simulink model "simulink"  (R2017a)
settings: Solver=ode5  StartTime=0.0  StopTime=inf  FixedStep=SampleTime  RelTol=1e-3  EnableMultiTasking=on
values from neighbouring files (symbols this model uses):
  max_velocity_1 = 14    [Matlab_script.m]
  max_velocity_2 = 15    [Matlab_script.m]
  max_velocity_3 = 13    [Matlab_script.m]
  max_velocity_4 = 100    [Matlab_script.m]
  SampleTime = 0.002    [Matlab_script.m]
  XY_vel = 0.5    [Matlab_script.m]
libraries: xpcrtudplib x2, etargetslib x1, xpcutilitieslib x1
settings Model: Creator=kivela6  LastModifiedBy=bangalor
settings SolverCC: EnableConcurrentExecution=on  ConcurrentTasks=on  AutoInsertRateTranBlk=on
settings DataIOCC: LimitDataPoints=on  SaveFormat=StructureWithTime  SignalLoggingSaveFormat=ModelDataLogs
settings OptimizationCC: BlockReduction=off  OptimizeBlockIOStorage=off  BufferReuse=off  GlobalBufferReuse=off  ExpressionFolding=off  EnableMemcpy=off  ExpressionDepthLimit=2147483647  LocalBlockOutputs=off
settings DebuggingCC: UnderspecifiedInitializationDetection=Classic  MergeDetectMultiDrivingBlocksExec=none  SolverPrmCheckMsg=warning  FcnCallInpInsideContextMsg=warning  StateNameClashWarn=warning  SFUnexpectedBacktrackingDiag=warning  SFNoUnconditionalDefaultTransitionDiag=warning  SFExecutionAtInitializationDiag=none
settings HardwareCC: ProdBitPerPointer=32  ProdBitPerSizeT=32  ProdBitPerPtrDiffT=32  ProdLargestAtomicFloat=None  ProdWordSize=32  ProdLongLongMode=on  ProdHWDeviceType=Generic->32-bit x86 compatible
settings ModelReferenceCC: PropagateSignalLabelsOutOfModel=off
settings RTWCC: SystemTargetFile=slrt.tlc  TemplateMakefile=slrt_default_tmf  Description=Simulink Real-Time  RTWCompilerOptimization=on
settings SimulinkRealTimeCC: xPCisDownloadable=off  xPCConcurrentTasks=on
settings ConfigComp: CovMetricSettings=dw  CovHtmlReporting=on  CovSaveCumulativeToWorkspaceVar=on  CovSaveSingleToWorkspaceVar=on  CovExternalEMLEnable=off  CovSFcnEnable=off

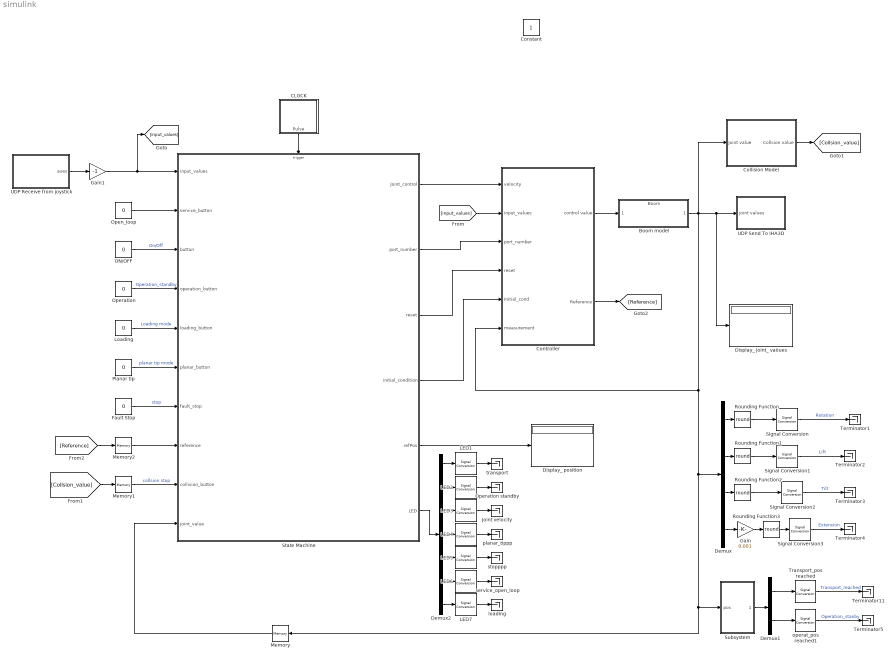
== system simulink ==
  Boom model : ModelReference  ModelNameDialog=Boom.slxp  ModelReferenceVersion=1.513  CopyOfModelProtected=on
  CLOCK : Subsystem
  Collision Model : Subsystem
  Controller : Subsystem
  Demux : Demux
  Demux1 : Demux  Outputs=2
  Demux2 : Demux  Outputs=7
  Display_ joint_ vaöues : Display
  Display_ position : Display
  Fault Stop : Constant  Value=0
  Gain : Gain  Gain=0.001
  Gain1 : Gain  Gain=-1
  Joint velocity : Terminator
  LED{1..7} (7 alike) : SignalConversion  OverrideOpt=off
  Loading : Constant  Value=0
  Memory : Memory
  Memory1 : Memory
  Memory2 : Memory
  ON/OFF : Constant  Value=0
  Open_loop : Constant  Value=0
  Operation : Constant  Value=0
  Operation standby : Terminator
  Planar tip : Constant  Value=0
  Rounding Function{,1..3} (4 alike) : Rounding  Operator=round
  Signal Conversion{,1..3} (4 alike) : SignalConversion  OverrideOpt=off
  State Machine : Stateflow chart  TreatAsAtomicUnit=on
  Subsystem : Subsystem
  Terminator{1..5,11} (6 alike) : Terminator
  Transport_pos reached : SignalConversion  OverrideOpt=off
  UDP Receive from joystick : Subsystem
  UDP Send To IHA3D : Subsystem
  loading : Terminator
  operat_pos reached1 : SignalConversion  OverrideOpt=off
  planar_tippp : Terminator
  service_open_loop : Terminator
  stopppp : Terminator
  transport : Terminator
  Constant : Constant  IOType=siggen
  wires:
  State Machine/1(Joint_control) -> Controller/1(velocity)
  CLOCK/1(Pulse) -> State Machine/Trigger
  Controller/1(control value) -> Boom model/1
  Memory/1 -> State Machine/10(joint_value)
  [input_values] -> Controller/2(input_values)
  State Machine/2(port_number) -> Controller/3(port_number)
  State Machine/3(reset) -> Controller/4(reset)
  State Machine/4(initial_condition) -> Controller/5(Initial_cond)
  Demux/1 -> Rounding Function/1
  Rounding Function/1 -> Signal Conversion/1
  Signal Conversion/1 -> Terminator1/1  "Rotation"
  Signal Conversion1/1 -> Terminator2/1  "Lift"
  Rounding Function1/1 -> Signal Conversion1/1
  Demux/2 -> Rounding Function1/1
  Demux/3 -> Rounding Function2/1
  Rounding Function2/1 -> Signal Conversion2/1
  Signal Conversion2/1 -> Terminator3/1  "Tilt"
  Signal Conversion3/1 -> Terminator4/1  "Extension"
  ON/OFF/1 -> State Machine/3(button)  "On/Off"
  Operation/1 -> State Machine/4(operation_button)  "Operation_standby"
  Loading/1 -> State Machine/5(loading_button)  "Loading mode"
  Planar tip/1 -> State Machine/6(planar_button)  "planar tip mode"
  Collision Model/1(Collsion value) -> [Collsion_value]
  UDP Receive from joystick/1(axes) -> Gain1/1
  Open_loop/1 -> State Machine/2(service_button)
  [Collsion_value] -> Memory1/1
  Fault Stop/1 -> State Machine/7(fault_stop)  "stop"
  Memory1/1 -> State Machine/9(collision_button)  "collsion stop"
  State Machine/5(refPos) -> Display_ position/1
  Demux1/2 -> operat_pos reached1/1
  Demux1/1 -> Transport_pos reached/1
  Boom model/1 -> Display_ joint_ vaöues/1, UDP Send To IHA3D/1(joint values), Controller/6(measurement), Memory/1, Subsystem/1(pos), Demux/1, Collision Model/1(Joint value)
  Subsystem/1(LED State) -> Demux1/1
  Transport_pos reached/1 -> Terminator11/1  "Transport_reached"
  State Machine/6(LED) -> Demux2/1
  Demux2/1 -> LED1/1
  LED1/1 -> transport/1
  LED2/1 -> Operation standby/1
  Demux2/2 -> LED2/1
  LED3/1 -> Joint velocity/1
  Demux2/3 -> LED3/1
  LED4/1 -> planar_tippp/1
  Demux2/4 -> LED4/1
  LED5/1 -> stopppp/1
  Demux2/5 -> LED5/1
  LED6/1 -> service_open_loop/1
  Demux2/6 -> LED6/1
  Demux2/7 -> LED7/1
  operat_pos reached1/1 -> Terminator5/1  "Operation_stanby"
  Controller/2(Reference) -> [Reference]
  [Reference] -> Memory2/1
  Memory2/1 -> State Machine/8(reference)
  LED7/1 -> loading/1
  Gain/1 -> Rounding Function3/1
  Rounding Function3/1 -> Signal Conversion3/1
  Demux/4 -> Gain/1
  Gain1/1 -> [input_values], State Machine/1(input_values)

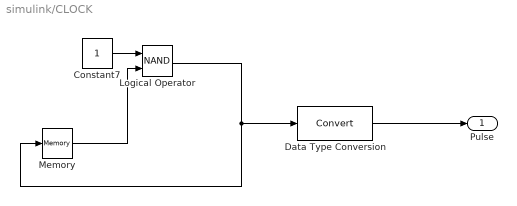
== system simulink/CLOCK ==
  Constant7 : Constant
  Data Type Conversion : DataTypeConversion
  Logical Operator : Logic  Operator=NAND  AllPortsSameDT=off  OutDataTypeStr=boolean
  Memory : Memory
  Pulse : Outport
  wires:
  Memory/1 -> Logical Operator/2
  Constant7/1 -> Logical Operator/1
  Logical Operator/1 -> Memory/1, Data Type Conversion/1
  Data Type Conversion/1 -> Pulse/1

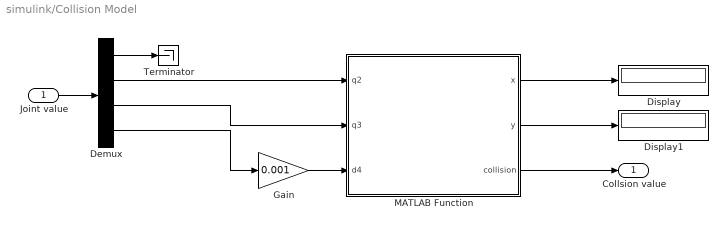
== system simulink/Collision Model ==
  Joint value : Inport
  Demux : Demux
  Display : Display
  Display1 : Display
  Gain : Gain  Gain=0.001
  MATLAB Function : MATLAB Function  TreatAsAtomicUnit=on
  Terminator : Terminator
  Collsion value : Outport
  wires:
  Demux/4 -> Gain/1
  MATLAB Function/2(y) -> Display1/1
  MATLAB Function/1(x) -> Display/1
  MATLAB Function/3(collision) -> Collsion value/1
  Demux/3 -> MATLAB Function/2(q3)
  Demux/2 -> MATLAB Function/1(q2)
  Demux/1 -> Terminator/1
  Joint value/1 -> Demux/1
  Gain/1 -> MATLAB Function/3(d4)

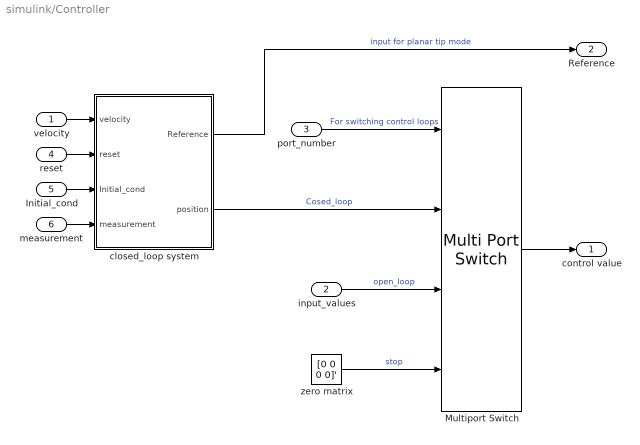
== system simulink/Controller ==
  velocity : Inport
  input_values : Inport  Port=2
  port_number : Inport  Port=3
  reset : Inport  Port=4
  Initial_cond : Inport  Port=5
  measurement : Inport  Port=6
  Multiport Switch : MultiPortSwitch  DiagnosticForDefault=Warning
  closed_loop system : Subsystem
  zero matrix : Constant  Value=[0 0 0 0]'
  control value : Outport
  Reference : Outport  Port=2
  wires:
  zero matrix/1 -> Multiport Switch/4  "stop"
  Multiport Switch/1 -> control value/1
  input_values/1 -> Multiport Switch/3  "open_loop"
  port_number/1 -> Multiport Switch/1  "For switching control loops"
  velocity/1 -> closed_loop system/1(velocity)
  reset/1 -> closed_loop system/2(reset)
  Initial_cond/1 -> closed_loop system/3(Initial_cond)
  measurement/1 -> closed_loop system/4(measurement)
  closed_loop system/1(Reference) -> Reference/1  "input for planar tip mode"
  closed_loop system/2(position) -> Multiport Switch/2  "Cosed_loop"

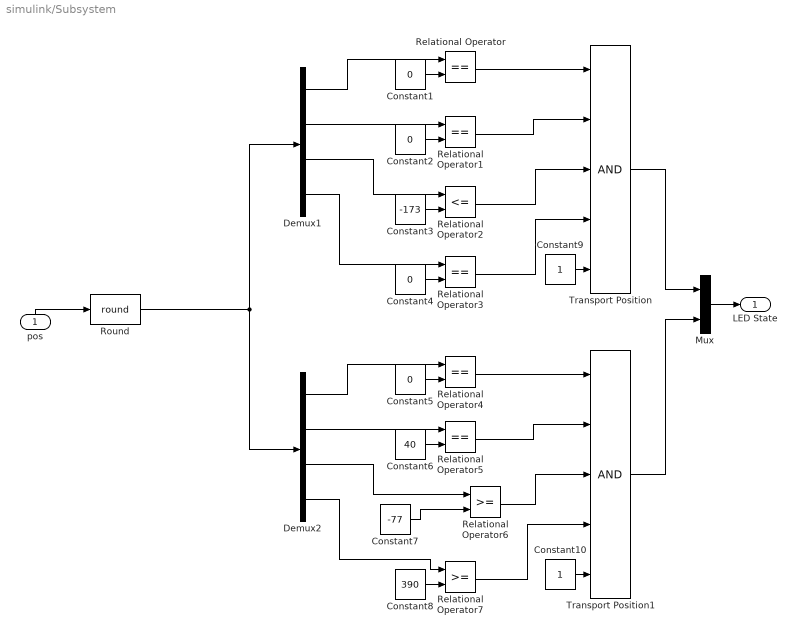
== system simulink/Subsystem ==
  pos : Inport
  Constant{1..2,4..5} (4 alike) : Constant  Value=0
  Constant10 : Constant
  Constant3 : Constant  Value=-173
  Constant6 : Constant  Value=40
  Constant7 : Constant  Value=-77
  Constant8 : Constant  Value=390
  Constant9 : Constant
  Demux1 : Demux
  Demux2 : Demux
  Mux : Mux  Inputs=2
  Relational Operator{,1,3..5} (5 alike) : RelationalOperator  Operator===  OutDataTypeStr=boolean  RndMeth=Simplest
  Relational Operator2 : RelationalOperator  Operator=<=  OutDataTypeStr=boolean  RndMeth=Simplest
  Relational Operator6 : RelationalOperator  OutDataTypeStr=boolean  RndMeth=Simplest
  Relational Operator7 : RelationalOperator  OutDataTypeStr=boolean  RndMeth=Simplest
  Round : Rounding  Operator=round
  Transport Position : Logic  Inputs=5  AllPortsSameDT=off  OutDataTypeStr=boolean
  Transport Position1 : Logic  Inputs=5  AllPortsSameDT=off  OutDataTypeStr=boolean
  LED State : Outport
  wires:
  Demux1/4 -> Relational Operator3/1
  Relational Operator3/1 -> Transport Position/4
  Constant4/1 -> Relational Operator3/2
  pos/1 -> Round/1
  Constant9/1 -> Transport Position/5
  Relational Operator4/1 -> Transport Position1/1
  Relational Operator5/1 -> Transport Position1/2
  Relational Operator7/1 -> Transport Position1/4
  Constant10/1 -> Transport Position1/5
  Relational Operator6/1 -> Transport Position1/3
  Relational Operator/1 -> Transport Position/1
  Constant1/1 -> Relational Operator/2
  Transport Position/1 -> Mux/1
  Relational Operator2/1 -> Transport Position/3
  Relational Operator1/1 -> Transport Position/2
  Demux2/1 -> Relational Operator4/1
  Demux2/2 -> Relational Operator5/1
  Constant8/1 -> Relational Operator7/2
  Demux2/3 -> Relational Operator6/1
  Constant5/1 -> Relational Operator4/2
  Constant6/1 -> Relational Operator5/2
  Demux2/4 -> Relational Operator7/1
  Constant2/1 -> Relational Operator1/2
  Constant3/1 -> Relational Operator2/2
  Demux1/3 -> Relational Operator2/1
  Demux1/2 -> Relational Operator1/1
  Demux1/1 -> Relational Operator/1
  Transport Position1/1 -> Mux/2
  Mux/1 -> LED State/1
  Round/1 -> Demux1/1, Demux2/1
  Constant7/1 -> Relational Operator6/2

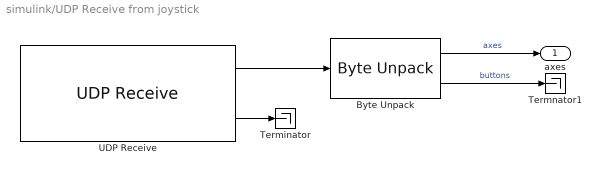
== system simulink/UDP Receive from joystick ==
  Byte Unpack : etargetslib/Byte Unpack  dimensions={4,12}  datatypes={'double','uint8'}  byteAlign=1
  Terminator : Terminator
  Termnator1 : Terminator
  UDP Receive : xpcrtudplib/UDP Receive  ipAddressVal=Use host-target connection  localPort=55550  rcvWidth=44  rcvFmAny=off  fmAddress=192.168.10.1  sampleTime=-1
      settings: SourceProductName=Simulink Real-Time
  axes : Outport
  wires:
  UDP Receive/2 -> Terminator/1
  UDP Receive/1 -> Byte Unpack/1
  Byte Unpack/1 -> axes/1  "axes"
  Byte Unpack/2 -> Termnator1/1  "buttons"

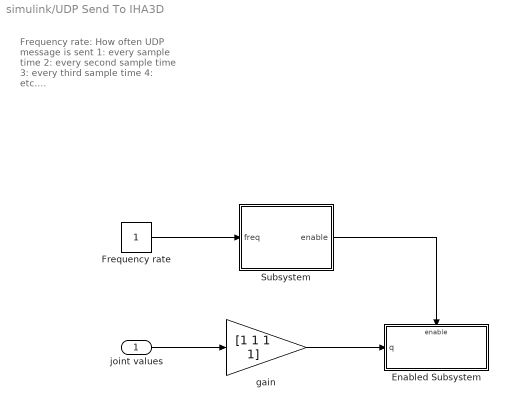
== system simulink/UDP Send To IHA3D ==
  note: Frequency rate:
      | How often UDP message is sent
      | 1: every sample time
      | 2: every second sample time
      | 3: every third sample time
      | 4: etc....
  joint values : Inport
  Enabled Subsystem : Subsystem  TreatAsAtomicUnit=on
  Frequency rate : Constant
  Subsystem : Subsystem
  gain : Gain  Gain=[1 1 1 1]
  wires:
  Subsystem/1(enable) -> Enabled Subsystem/Enable
  Frequency rate/1 -> Subsystem/1(freq)
  joint values/1 -> gain/1
  gain/1 -> Enabled Subsystem/1(q)

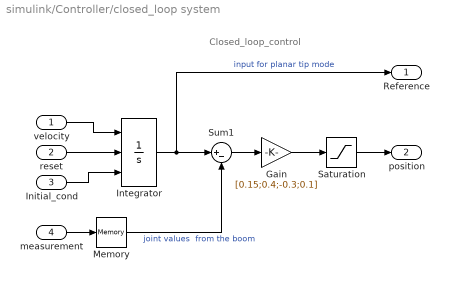
== system simulink/Controller/closed_loop system ==
  note: Closed_loop_control
  velocity : Inport
  reset : Inport  Port=2
  Initial_cond : Inport  Port=3
  measurement : Inport  Port=4
  Gain : Gain  Gain=[0.15;0.4;-0.3;0.1]
  Integrator : Integrator  ExternalReset=either  InitialConditionSource=external  LimitOutput=on  UpperSaturationLimit=[140;75;-10;1800]  LowerSaturationLimit=[-140;0;-175;0]
  Memory : Memory
  Saturation : Saturate  UpperLimit=1  LowerLimit=-1
  Sum1 : Sum  Inputs=|+-
  Reference : Outport
  position : Outport  Port=2
  wires:
  measurement/1 -> Memory/1
  Gain/1 -> Saturation/1
  Sum1/1 -> Gain/1
  velocity/1 -> Integrator/1
  Memory/1 -> Sum1/2  "joint values  from the boom"
  Integrator/1 -> Reference/1, Sum1/1  "input for planar tip mode"
  Saturation/1 -> position/1
  reset/1 -> Integrator/2
  Initial_cond/1 -> Integrator/3

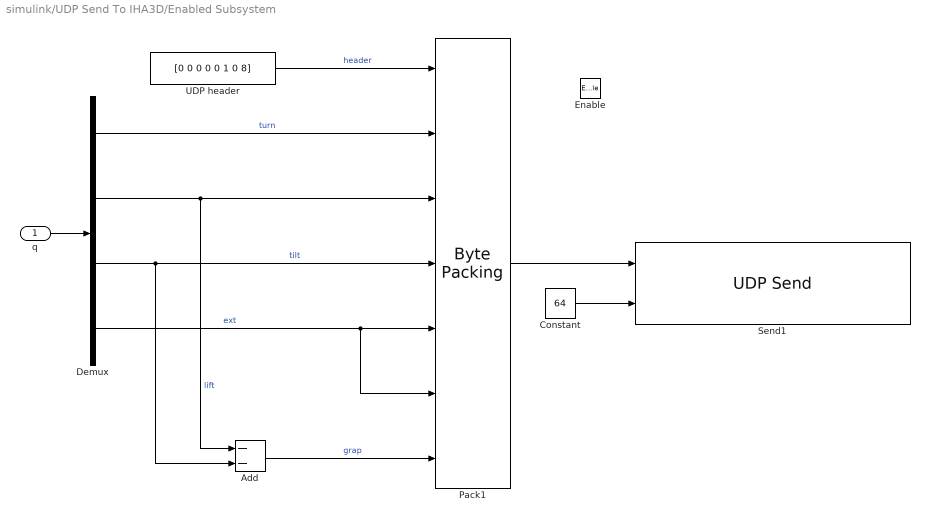
== system simulink/UDP Send To IHA3D/Enabled Subsystem ==
  q : Inport
  Enable : EnablePort
  Add : Sum  Inputs=--
  Constant : Constant  Value=64
  Demux : Demux
  Pack1 : xpcutilitieslib/Byte Packing   MaskPackedDataType=uint8  MaskUnpackedDataTypes={'uint8','double','double','double','double','double','double'}  MaskAlignment=1
  Send1 : xpcrtudplib/UDP Send  ipAddressVal=Use host-target connection  localPort=5555  toAddress=192.168.10.1  toPort=7755  sampleTime=SampleTime
      settings: SourceProductName=Simulink Real-Time  SourceProductBaseCode=XP
  UDP header : Constant  Value=[0 0 0 0 0 1 0 8]  OutDataTypeStr=uint8
  wires:
  UDP header/1 -> Pack1/1  "header"
  q/1 -> Demux/1
  Demux/2 -> Pack1/3, Add/1  "lift"
  Demux/3 -> Pack1/4, Add/2  "tilt"
  Demux/4 -> Pack1/6, Pack1/5  "ext"
  Add/1 -> Pack1/7  "grap"
  Demux/1 -> Pack1/2  "turn"
  Pack1/1 -> Send1/1
  Constant/1 -> Send1/2

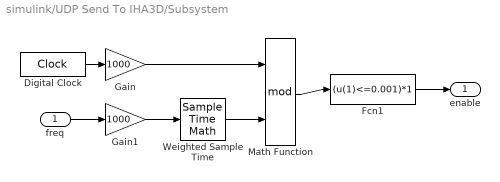
== system simulink/UDP Send To IHA3D/Subsystem ==
  freq : Inport
  Digital Clock : DigitalClock  SampleTime=SampleTime
  Fcn1 : Fcn  Expr=(u(1)<=0.001)*1
  Gain : Gain  Gain=1000
  Gain1 : Gain  Gain=1000  SampleTime=SampleTime
  Math Function : Math  Operator=mod  SaturateOnIntegerOverflow=on
  Weighted Sample Time : SampleTimeMath  TsampMathOp=*
  enable : Outport
  wires:
  Weighted Sample Time/1 -> Math Function/2
  freq/1 -> Gain1/1
  Math Function/1 -> Fcn1/1
  Gain/1 -> Math Function/1
  Gain1/1 -> Weighted Sample Time/1
  Fcn1/1 -> enable/1
  Digital Clock/1 -> Gain/1

== matlab function simulink/Collision Model/MATLAB Function ==
  data: x output; q2 input; y output; q3 input; d4 input; collision output
function [x,y,collision] = FK(q2,q3,d4)
%#codegen

% This function transforms measured joint positions to the position of the
% Tool Center Point. In this case, the TCP is located at the end of the
% boom, after the telesopic joint and before the passive joint.
%
% The first joint angle, q1, has no effect on the kinematics, so it is not
% a part of this function.
%
% Inputs:
%   q2,q3,d4    - Current joint positions [deg,m]
%
% Outputs:
%   x,y         - Current TCP position position [m]
%

% YOU MAY NEED TO CHANGE THE FUNCTION CALL IF YOU CANNOT USE IT AS-IS.
% FOR EXAMPLE, YOU MAY NEED TO READ INPUTS FROM WORKSPACE VARIABLES HERE
% AT THE VERY BEGINNING OF THIS SCRIPT, AND THEN WRITE THE RESULTS TO
% WORKSPACE VARIABLES AT THE VERY END OF THIS SCRIPT.


% Unit conversion to radians and meters
deg_to_rad = pi/180;
q2 = q2*deg_to_rad;
q3 = q3*deg_to_rad;

% Calculate the forward kinematics
t1 = cos(q2);
t2 = q3 + pi / 0.2e1;
t3 = cos(t2);
t4 = sin(q2);
t2 = sin(t2);
t5 = t1 * t2 + t3 * t4;
t6 = d4 + 0.213e1;
t7 = 0.376348799999999983e0;
t8 = 0.350440540000000000e1;
t2 = t1 * t3 - t2 * t4;
t3 = 0.160450000000000004e1;
XY_kin = [t1 * t8 + t5 * t6 + t7 * t2 - 0.208160000000000012e0 -t2 * t6 + t4 * t8 + t5 * t7 + t3];

% Write results to outputs (in meters)
x = XY_kin(1);
y = XY_kin(2);



if x < 1.1
    collision =1; 
else
    collision = 0;
end
disp(collision)
end

== stateflow chart simulink/State Machine ==
  state Off									% Machine Off State
    entry:
    LED = [0;0;0;0;0;0;0];				% LED status of User Interface
    Joint_control = [0;0;0;0];
    reset = 1;							%reset value to controller integrator
    initial_condition = joint_value;		% initial condition to controller integrator
  state On % Machine On state
    state Transport_Position_state					% to move boom to transport position
      entry:
      initial_condition = joint_value;				% initial condition to controller integrator
      Joint_control =[0;0;0;0];
      port_number = 1;
      state Automatic_movement				%function for automatic movement
        entry:
        LED = [1;0;0;0;0;0;0];				% LED status of User Interface
        port_number = 1;					% to choose closed loop control in the controller
        refPos = joint_value;				% joint position value to verify during automatic mode
        fla_g = 0;							% flag variable used in function as output
        during:
        reset = 1;							%reset value to controller integrator
        [Joint_control,refPos,fla_g]= tg([0;0;-175;0], joint_value, input_values(2)*1.05);		% function for the automatic control of boom to target position
        exit:
        reset =1;
      (default) -> On.Transport_Position_state.Automatic_movement				%function for automatic movement
    state Service_Mode									% to operate teh system in open loop control
      entry:
      LED = [0;0;0;0;0;1;0];							% LED status of User Interface
      Joint_control = [0;0;0;0];
      port_number = 3;								% to choose to stop in the controller
      during:
      port_number = 2;								% to choose open loop control during action in the controller
      Joint_control = (input_values/2);
      exit:
      port_number = 1;								% to choose teh close loop control during exit
      initial_condition = joint_value;					% initial condition to controller integrator
      reset = reset-1;
    state operation_stanby_state					% to move boom to operation standby position
      entry:
      initial_condition = joint_value;				% initial condition to controller integrator
      Joint_control =[0;0;0;0];
      port_number = 1;
      state Automatic_movement				%function for automatic movement
        entry:
        LED = [0;1;0;0;0;0;0];				% LED status of User Interface
        port_number = 1;					% to choose closed loop control in the controller
        refPos = joint_value;				% joint position value to verify during automatic mode
        fla_g = 0;							% flag variable used in function as output
        during:
        reset = 1;							%reset value to controller integrator
        [Joint_control,refPos,fla_g]= tg([0;40;-75;400], joint_value, input_values(2));  	% function for the automatic control of boom to target position
        exit:
        reset = 1;
      (default) -> On.operation_stanby_state.Automatic_movement				%function for automatic movement
    state loading_mode
      entry:
      state Joint_velocity_mode												% Joint control of joints separaetly
        entry:
        LED = [0;0;1;0;0;0;1];												% LED status of User Interface
        Joint_control = [0;0;0;0];
        initial_condition = joint_value;										% initial condition as joint value to controller integrator
        reset = 1;															%reset value to controller integrator
        port_number = 1;													% to choose closed loop control in the controller
        during:
        Joint_control(1)=input_values(1)*max_velocity_1;				% joint control by joystick input values for respective joints
        Joint_control(2)=input_values(2)*max_velocity_2;				% joystick input is multiplied by gain to improve the speed of boom
        Joint_control(3)=input_values(3)*max_velocity_3;
        Joint_control(4)=input_values(4)*max_velocity_4;
      state Planar_tip_mode							% boom tip control in planar co-ordiante axis
        entry:
        LED = [0;0;0;1;0;0;1];						% LED status of User Interface
        Joint_control = [0;0;0;0];
        initial_condition = joint_value;
        reset= 1;
        port_number = 1;							% to choose closed loop control in the controller
        during:
        % control of q2,q3, d4 by only input of joystick axes 2 and 3. Inverse Kinematics matlab function is used for the planar tip movement
        [Joint_control(2),Joint_control(3),Joint_control(4)] = IK_vel(reference(2),reference(3),reference(4),input_values(2)*XY_vel,input_values(3)*XY_vel);
        Joint_control(1) = input_values(1)*max_velocity_1;				% control of q1 by input axis (1)
      (default) -> Joint_velocity_mode												% Joint control of joints separaetly
      Joint_velocity_mode												% Joint control of joints separaetly -> Planar_tip_mode							% boom tip control in planar co-ordiante axis : [planar_button == 1]
      Planar_tip_mode							% boom tip control in planar co-ordiante axis -> Joint_velocity_mode												% Joint control of joints separaetly : [planar_button == 0]
    state Collision_mode					% to stop whne collision is deteced
      entry:
      LED = [0;0;0;0;1;0;0];				% LED status of User Interface
      Joint_control = [0;0;0;0];
      port_number = 3;					% to choose closed loop control in the controller
    (default) -> Transport_Position_state					% to move boom to transport position
    Service_Mode									% to operate teh system in open loop control -> Transport_Position_state					% to move boom to transport position : [service_button == 0]
    loading_mode -> Service_Mode									% to operate teh system in open loop control [order 1] : [service_button == 1]
    Transport_Position_state					% to move boom to transport position -> Service_Mode									% to operate teh system in open loop control [order 3] : [service_button == 1]
    operation_stanby_state					% to move boom to operation standby position -> Service_Mode									% to operate teh system in open loop control [order 2] : [service_button == 1]
    Transport_Position_state					% to move boom to transport position -> Collision_mode					% to stop whne collision is deteced [order 1] : [collision_button == 1]
    Transport_Position_state					% to move boom to transport position -> operation_stanby_state					% to move boom to operation standby position [order 2] : [operation_button == 1]
    operation_stanby_state					% to move boom to operation standby position -> Transport_Position_state					% to move boom to transport position [order 1] : [operation_button == 0]
    Collision_mode					% to stop whne collision is deteced -> Service_Mode									% to operate teh system in open loop control : [service_button == 1]
    operation_stanby_state					% to move boom to operation standby position -> Collision_mode					% to stop whne collision is deteced [order 4] : [collision_button == 1]
    operation_stanby_state					% to move boom to operation standby position -> loading_mode [order 3] : [loading_button == 1]
    loading_mode -> operation_stanby_state					% to move boom to operation standby position [order 3] : [loading_button == 0]
    loading_mode -> Collision_mode					% to stop whne collision is deteced [order 2] : [collision_button == 1]
  state Safe_state_stop				% Safe stop mode for Emergency STOP
    entry:
    LED = [0;0;0;0;1;0;0];			% LED status of User Interface
    Joint_control = [0;0;0;0];
    port_number = 3;				%to stop all the boom movements in controller
  (default) -> Off									% Machine Off State
  Off									% Machine Off State -> On % Machine On state : [button == 1]
  On % Machine On state -> Off									% Machine Off State [order 1] : [button == 0]
  On % Machine On state -> Safe_state_stop				% Safe stop mode for Emergency STOP [order 2] : [fault_stop == 1]
  Safe_state_stop				% Safe stop mode for Emergency STOP -> On % Machine On state : [fault_stop == 0]
  data: v function_output; p function_output; pt function_input; pmea function_input; cont function_input; flag function_output; q2 function_input; q3 function_input; d4 function_input; xvel function_input; yvel function_input; q2vel function_output; q3vel function_output; d4vel function_output; input_values input; service_button input; button input; Joint_control output; operation_button input; loading_button input; planar_button input; max_velocity_1 parameter double; fault_stop input; reference input; collision_button input; joint_value input; port_number output; reset output; fla_g local; initial_condition output; XY_vel parameter; refPos output; LED output; max_velocity_2 parameter double; max_velocity_3 parameter double; max_velocity_4 parameter double
  events: clock input EITHER_EDGE_EVENT
  function [v,p,flag]= tg(pt,pmea,cont):
    | function [v,p,flag]= tg(pt,pmea,cont)       %pt - target position
    | dt = 0.01;
    | cont = abs(cont);                   %cont - joystick input value
    | v=zeros(4,1);
    | dist=(pt-pmea);
    | %t=2.3;
    | t = 3.2;                         % assuming the average time for operation
    | v= cont*(dist/t);                %joystick Input*averageVelocity 
    | p= pmea+v*dt;
    | flag=0;
    | end
  function [q2vel,q3vel,d4vel] = IK_vel(q2,q3,d4,xvel,yvel):
    | function [q2vel,q3vel,d4vel] = IK_vel(q2,q3,d4,xvel,yvel)
    | %#codegen
    | 
    | % This function transforms desired coordinate velocities to desired joint
    | % velocities in such a way that the joints move as little as possible. To
    | % do this, the function needs to also know the current pose (joint
    | % positions) of the manipulator.
    | %
    | % Notice that the output is a set of desired joint velocities, not
    | % absolute joint positions. If you know the discrete time step you are
    | % using, you can integrate those velocities into a change of position.
    | %
    | % Likewise, the inputs xvel & yvel are desired coordinate velocities, not
    | % desired absolute coordinate positions. If you want to explicitly control
    | % coordinate positions, you can calculate the time derivative of your
    | % desired coordinate positions to get the desired velocities.
    | %
    | % The first joint angle, q1, has no effect on the kinematics, so it is not
    | % a part of this function.
    | %
    | % Inputs:
    | %   q2,q3,d4            - Current joint position references
    | %                         e.g. from last iteration [deg,m]
    | %   xvel,yvel           - Desired coordinate velocities [m/s]
    | %
    | % Outputs:
    | %   q2vel,q3vel,d4vel   - Desired joint velocities [deg/s,m/s]
    | %
    | 
    | 
    | % YOU MAY NEED TO CHANGE THE FUNCTION CALL IF YOU CANNOT USE IT AS-IS.
    | % FOR EXAMPLE, YOU MAY NEED TO READ INPUTS FROM WORKSPACE VARIABLES HERE
    | % AT THE VERY BEGINNING OF THIS SCRIPT, AND THEN WRITE THE RESULTS TO
    | % WORKSPACE VARIABLES AT THE VERY END OF THIS SCRIPT.
    | 
    | 
    | % Unit conversion to radians and meters
    | deg_to_rad = pi/180;
    | rad_to_deg = 180/pi;
    | q2 = q2*deg_to_rad;
    | q3 = q3*deg_to_rad;
    | d4 = d4/1000;
    | 
    | % Calculate the [3*2] Jacobian pseudoinverse
    | t1 = sin(q2);
    | t2 = q3 + pi / 0.2e1;
    | t3 = cos(t2);
    | t4 = cos(q2);
    | t2 = sin(t2);
    | t5 = -t1 * t2 + t3 * t4;
    | t6 = d4 + 0.213e1;
    | t7 = t4 * t2;
    | t8 = t1 * t3;
    | t9 = t7 + t8;
    | t10 = 0.350440540000000000e1;
    | t11 = t9 * 0.376348799999999983e0;
    | t12 = t5 * t6;
    | t13 = -t1 * t10 - t11 + t12;
    | t14 = t1 ^ 2;
    | t15 = t14 ^ 2;
    | t16 = t4 ^ 2;
    | t17 = t16 ^ 2;
    | t18 = t3 ^ 2;
    | t19 = t18 ^ 2;
    | t20 = t7 * t1;
    | t21 = t1 * t18 * t4;
    | t22 = d4 * (t2 * (t3 * (-t16 + t14) + t20) - t21);
    | t23 = t4 * t9;
    | t24 = t2 ^ 2;
    | t25 = t24 ^ 2;
    | t26 = t14 * t18 + t16 * t24;
    | t27 = d4 ^ 2;
    | t28 = -t16 + t14;
    | t29 = t3 * t28;
    | t30 = t2 * (t20 + t29) - t21;
    | t31 = t14 * t24 + t16 * t18;
    | t32 = 0.1492876700e2;
    | t33 = 0.7008810800e1;
    | t34 = 0.2637757534e1;
    | t35 = 0.1283276839e1;
    | t36 = 0.8520000000e1;
    | t37 = 0.9073800000e1;
    | t38 = (0.4e1 * d4 + 0.1704000000e2) * d4;
    | t39 = 0.1505395200e1 * t22;
    | t40 = 0.3206491776e1 * t30;
    | t8 = d4 * t23 * t33 + d4 * t26 * t36 + t34 * t4 * t5 + t23 * t32 + 0.2e1 * t27 * t26 + t26 * t37 + t31 * t35 + t4 * (0.1228085721e2 * t4 + t8 * t2 * (t38 + 0.1558104632e2)) - t39 - t40;
    | t23 = t18 + t24;
    | t23 = t2 * (t15 * t23 + t17 * t23);
    | t41 = t18 + t24;
    | t42 = t14 * t16;
    | t43 = t42 * t2;
    | t44 = t17 + t15;
    | t45 = t3 * t2;
    | t46 = t42 * t24;
    | t47 = t42 * t19;
    | t48 = t24 * (t18 * (t17 + t15) + t46) + t47;
    | t49 = t18 * t44;
    | t50 = t19 + t25;
    | t50 = t15 * t50 + t17 * t50;
    | t19 = t19 + t25;
    | t25 = 0.9073800003e1;
    | t51 = 0.1814760000e2;
    | t15 = d4 * t23 * t33 + 0.1401762160e2 * t43 * d4 * t41 - 0.9243771744e1 * t45 * d4 * t44 + 0.2985753400e2 * t43 * t41 + 0.5231645170e2 * t49 * d4 - 0.1968923382e2 * t45 * t44 + 0.1228085721e2 * t49 * t27 + t51 * (t24 * (t46 + t49) + t47) + 0.8519999996e1 * d4 * t50 + t23 * t32 + t25 * (t15 * t19 + t17 * t19) + 0.1402029841e2 * t24 * t44 + 0.5571702104e2 * t49 + 0.1704000000e2 * d4 * t48 + 0.4e1 * t27 * t48 + 0.2e1 * t27 * t50 + t42 * (t3 * (t2 * (-0.1848754340e2 * d4 - 0.3937846770e2) + t3 * (((0.8e1 * t24 + 0.2456171442e2) * d4 + 0.3408000000e2 * t24 + 0.1046329034e3) * d4 + 0.3629520000e2 * t24 + 0.1114340422e3)) + 0.2804059680e2 * t24);
    | t17 = t5 * 0.376348799999999983e0;
    | t6 = t9 * t6;
    | t10 = t10 * t4 + t17 + t6;
    | t19 = t18 - t24;
    | t23 = 0.1603245888e1;
    | t2 = t22 * t36 + 0.7790523161e1 * t30 + 0.3504405400e1 * t29 * d4 - 0.7526976000e0 * d4 * (t14 * (-t18 + t24) + t16 * (t18 - t24)) + 0.7464383502e1 * t29 - 0.1318878767e1 * t2 * t28 + t23 * (t14 * t19 - t16 * t19) - 0.2e1 * t27 * (t2 * (t3 * (t16 - t14) - t20) + t21) + t1 * t4 * (t2 * (d4 * t33 + t3 * (0.3010790400e1 * d4 + 0.6412983552e1) + t32) + t3 * t34 + 0.1228085721e2);
    | t4 = 0.1e1 / t15;
    | t14 = t1 * t5;
    | t1 = -t33 * t14 * d4 + t36 * d4 * t31 + t34 * t1 * t9 + t1 * (0.1228085721e2 * t1 + t7 * t3 * (-t38 - 0.1558104632e2)) - t14 * t32 + t26 * t35 + 0.2e1 * t27 * t31 + t31 * t37 + t39 + t40;
    | t3 = t12 - t11;
    | t6 = t6 + t17;
    | Jacob_pinv = [t4 * (t10 * t2 + t13 * t8) t4 * (t1 * t10 + t13 * t2); t4 * (t2 * t6 + t3 * t8) t4 * (t1 * t6 + t3 * t2); t4 * (-t2 * t5 + t8 * t9) t4 * (-t1 * t5 + t2 * t9);];
    | 
    | % Use the pseudoinverse to calculate the desired joint velocities
    | IK_result = Jacob_pinv * [xvel yvel]';
    | 
    | % Write results to outputs, with unit conversion to deg/s and mm/s
    | q2vel = IK_result(1) * rad_to_deg;
    | q3vel = IK_result(2) * rad_to_deg;
    | d4vel = IK_result(3) * 1000;
    | 
    | 
    | % Limit output to prevent infinity values
    | if abs(q2vel) > 1000
    |     q2vel = sign(q2vel)*1000;
    | end
    | if abs(q3vel) > 1000
    |     q3vel = sign(q3vel)*1000;
    | end
    | if abs(d4vel) > 10000
    |     d4vel = sign(d4vel)*1000;
    | end
    | 
    | end
